simulink model "integrate_and_dump_multisignal_Team6"  (R2014a)
settings: Solver=ode45  StartTime=0.0  StopTime=10000  RelTol=1e-3
libraries: commfilt2 x4, commnoisgen2 x1
settings Model: Creator=alexw  LastModifiedBy=Renato
settings DataIOCC: SignalLoggingSaveFormat=ModelDataLogs
settings OptimizationCC: ExpressionDepthLimit=2147483647
settings DebuggingCC: UnderspecifiedInitializationDetection=Classic  FcnCallInpInsideContextMsg=UseLocalSettings  StateNameClashWarn=warning
settings GRTTargetCC: CombineOutputUpdateFcns=off  GRTInterface=on

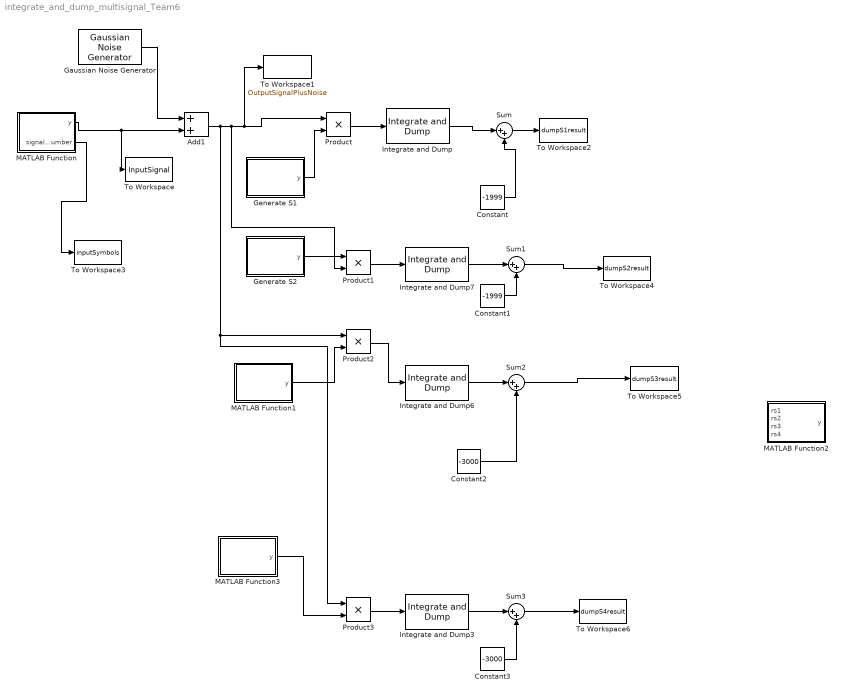
== system integrate_and_dump_multisignal_Team6 ==
  Add1 : Sum
  Constant : Constant  Value=-1999
  Constant1 : Constant  Value=-1999
  Constant2 : Constant  Value=-3000
  Constant3 : Constant  Value=-3000
  Gaussian Noise Generator : commnoisgen2/Gaussian Noise Generator  m=0  d=0.1  s=41  Ts=0.01  frameBased=on  sampPerFrame=3000  orient=off  outDataType=double
  "Generate S1 " : MATLAB Function  TreatAsAtomicUnit=on
  Generate S2 : MATLAB Function  TreatAsAtomicUnit=on
  Integrate and Dump{,3,6..7} (4 alike) : commfilt2/Integrate and Dump  obssamples=3000  offsetsamples=0  nodump=off  roundingMode=Floor  overflowMode=off
  MATLAB Function : MATLAB Function  TreatAsAtomicUnit=on
  MATLAB Function1 : MATLAB Function  TreatAsAtomicUnit=on
  MATLAB Function2 : MATLAB Function  TreatAsAtomicUnit=on
  MATLAB Function3 : MATLAB Function  TreatAsAtomicUnit=on
  Product{,1..3} (4 alike) : Product
  Sum{,1..3} (4 alike) : Sum  Inputs=|++
  To Workspace : ToWorkspace  VariableName=InputSignal  SampleTime=-1
      settings: Save2DSignal=2-D array (concatenate along first dimension)
  To Workspace1 : ToWorkspace  VariableName=OutputSignalPlusNoise  SampleTime=-1
      settings: Save2DSignal=2-D array (concatenate along first dimension)
  To Workspace2 : ToWorkspace  VariableName=dumpS1result  SampleTime=-1
      settings: Save2DSignal=2-D array (concatenate along first dimension)
  To Workspace3 : ToWorkspace  VariableName=inputSymbols  SampleTime=-1
      settings: Save2DSignal=2-D array (concatenate along first dimension)
  To Workspace4 : ToWorkspace  VariableName=dumpS2result  SampleTime=-1
      settings: Save2DSignal=2-D array (concatenate along first dimension)
  To Workspace5 : ToWorkspace  VariableName=dumpS3result  SampleTime=-1
      settings: Save2DSignal=2-D array (concatenate along first dimension)
  To Workspace6 : ToWorkspace  VariableName=dumpS4result  SampleTime=-1
      settings: Save2DSignal=2-D array (concatenate along first dimension)
  wires:
  MATLAB Function/1(y) -> To Workspace/1, Add1/2
  Gaussian Noise Generator/1 -> Add1/1
  "Generate S1 "/1(y) -> Product/2
  Add1/1 -> Product3/1, Product2/1, Product1/1, To Workspace1/1, Product/1
  Generate S2/1(y) -> Product1/2
  MATLAB Function1/1(y) -> Product2/2
  MATLAB Function3/1(y) -> Product3/2
  Product3/1 -> Integrate and Dump3/1
  Product2/1 -> Integrate and Dump6/1
  Product1/1 -> Integrate and Dump7/1
  Product/1 -> Integrate and Dump/1
  Integrate and Dump/1 -> Sum/1
  Constant/1 -> Sum/2
  Integrate and Dump7/1 -> Sum1/1
  Constant1/1 -> Sum1/2
  Integrate and Dump6/1 -> Sum2/1
  Constant2/1 -> Sum2/2
  Integrate and Dump3/1 -> Sum3/1
  Constant3/1 -> Sum3/2
  Sum/1 -> To Workspace2/1
  MATLAB Function/2(signalNumber) -> To Workspace3/1
  Sum3/1 -> To Workspace6/1
  Sum2/1 -> To Workspace5/1
  Sum1/1 -> To Workspace4/1

== matlab function integrate_and_dump_multisignal_Team6/MATLAB Function1 ==
  data: y output size=3000
function y = generateS3()
%#codegen
sampleRate = 1000;
time = linspace(0,3,3*sampleRate);
nsamples = length(time);



s3 = ones(1,nsamples);
s3(1:(2*sampleRate)-1) = 1;
s3(2*sampleRate:end) = -1;




y = s3';

== matlab function integrate_and_dump_multisignal_Team6/MATLAB Function ==
  data: y output size=3000; signalNumber output
function [y,signalNumber] = generateSingal
%#codegen
sampleRate = 1000;
time = linspace(0,3,3*sampleRate);
nsamples = length(time);

s1 = ones(1,nsamples);
s1(2*sampleRate:end) = 0;
tempInput = s1';
s2 = ones(1,nsamples);
s2(1:sampleRate-1) = 1;
s2(sampleRate:(2*sampleRate)-1) = -1;
s2(2*sampleRate:end) = 0;

s3 = ones(1,nsamples);
s3(1:(2*sampleRate)-1) = 1;
s3(2*sampleRate:end) = -1;


s4 = -1*ones(1,nsamples);

nextSignal = randi(4);
  
   
    switch nextSignal
        case 1
            tempInput = s1';
            
        case 2
            tempInput = s2';
            
        case 3
            tempInput = s3';
            
        case 4
            tempInput= s4';
            
    end
signalNumber = nextSignal;
y = tempInput;

== matlab function integrate_and_dump_multisignal_Team6/Generate S2 ==
  data: y output size=3000
function y = generateSingal()
%#codegen
sampleRate = 1000;
time = linspace(0,3,3*sampleRate);
nsamples = length(time);


s2 = ones(1,nsamples);
s2(1:sampleRate-1) = 1;
s2(sampleRate:(2*sampleRate)-1) = -1;
s2(2*sampleRate:end) = 0;

y = s2';

== matlab function integrate_and_dump_multisignal_Team6/MATLAB Function3 ==
  data: y output size=3000
function y = generateS4()
%#codegen
sampleRate = 1000;
time = linspace(0,3,3*sampleRate);
nsamples = length(time);

s4 = -1*ones(1,nsamples);



y = s4';

== matlab function integrate_and_dump_multisignal_Team6/Generate S1  ==
  data: y output size=3000
function y = generateS1()
%#codegen
sampleRate = 1000;
time = linspace(0,3,3*sampleRate);
nsamples = length(time);

s1 = ones(1,nsamples);
s1(2*sampleRate:end) = 0;
y = s1';

== matlab function integrate_and_dump_multisignal_Team6/MATLAB Function2 ==
  data: rs1 input; y output; rs2 input; rs3 input; rs4 input
function y = fcn(rs1,rs2,rs3,rs4)

%#codegen
temp = [ rs1, rs2,rs3,rs4];
[C index] = max(temp);
y = index;
